simulink subsystem "algebraic_PIO_observer"  (R2024a)
settings: Solver=VariableStepAuto  StartTime=0.0  StopTime=10.0  RelTol=1e-3
undefined symbols (not defined in the file): Af, Cd, g, h, kf_A, kf_B, kf_C, kf_D, kf_L, l, lf, lr, M, re, rho_air
settings Model: Creator=Henrique Mesquita  LastModifiedBy=Henrique Mesquita
settings DebuggingCC: UnconnectedInputMsg=warning  UnconnectedOutputMsg=warning  UnconnectedLineMsg=warning
settings ModelReferenceCC: EnableRefExpFcnMdlSchedulingChecks=on
settings RTWCC: GPUComputeCapability=3.5  DLArmComputeVersion=19.05

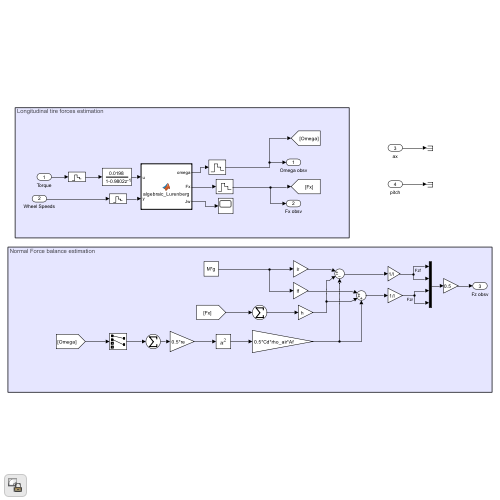
[thumbnail: Simulink's stored preview of the top-level diagram]
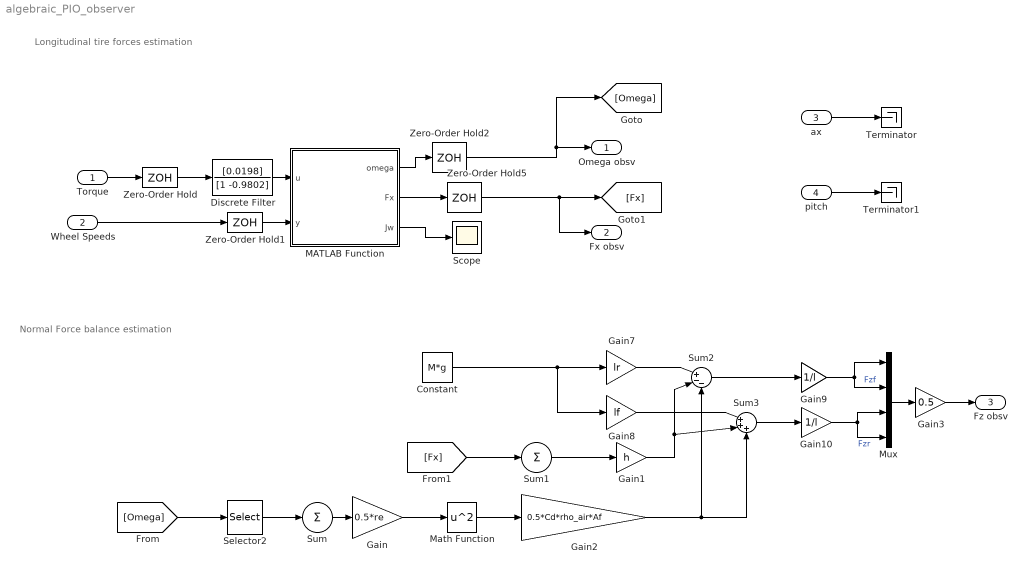
== system algebraic_PIO_observer ==
  note: Longitudinal tire forces estimation
  note: Normal Force balance estimation
  Torque : Inport  PortDimensions=4
  Wheel Speeds : Inport  Port=2  PortDimensions=4
  ax : Inport  Port=3  PortDimensions=1
  pitch : Inport  Port=4  PortDimensions=1
  Constant : Constant  Value=M*g
  Discrete Filter : DiscreteFilter  Numerator=[0.0198]  Denominator=[1 -0.9802]  SampleTime=0.001
  Gain : Gain  Gain=0.5*re
  Gain1 : Gain  Gain=h
  Gain10 : Gain  Gain=1/l
  Gain2 : Gain  Gain=0.5*Cd*rho_air*Af
  Gain3 : Gain  Gain=0.5
  Gain7 : Gain  Gain=lr
  Gain8 : Gain  Gain=lf
  Gain9 : Gain  Gain=1/l
  MATLAB Function : MATLAB Function  TreatAsAtomicUnit=on
  Math Function : Math  Operator=square
  Mux : Mux
  Scope : Scope
  Selector2 : Selector  InputPortWidth=4  IndexOptions=Index vector (dialog)  Indices=[1 2]  OutputSizes=1
  Sum : Sum  Inputs=+
  Sum1 : Sum  Inputs=+
  Sum2 : Sum  Inputs=|+--
  Sum3 : Sum  Inputs=|+++
  Terminator : Terminator
  Terminator1 : Terminator
  Zero-Order Hold{,1..2,5} (4 alike) : ZeroOrderHold  SampleTime=0.001
  Omega obsv : Outport
  Fx obsv : Outport  Port=2
  Fz obsv : Outport  Port=3
  wires:
  [Omega] -> Selector2/1
  Discrete Filter/1 -> MATLAB Function/1(u)
  Mux/1 -> Gain3/1
  Gain9/1 -> Mux/1, Mux/2  "Fzf"
  Gain2/1 -> Sum2/3, Sum3/3
  Gain1/1 -> Sum2/2, Sum3/2
  Gain3/1 -> Fz obsv/1
  Torque/1 -> Zero-Order Hold/1
  Constant/1 -> Gain7/1, Gain8/1
  Zero-Order Hold/1 -> Discrete Filter/1
  Gain/1 -> Math Function/1
  Math Function/1 -> Gain2/1
  Selector2/1 -> Sum/1
  [Fx] -> Sum1/1
  Gain7/1 -> Sum2/1
  Sum3/1 -> Gain10/1
  Gain10/1 -> Mux/3, Mux/4  "Fzr"
  MATLAB Function/1(omega) -> Zero-Order Hold2/1
  Zero-Order Hold2/1 -> Omega obsv/1, [Omega]
  Zero-Order Hold1/1 -> MATLAB Function/2(y)
  pitch/1 -> Terminator1/1
  Zero-Order Hold5/1 -> [Fx], Fx obsv/1
  Wheel Speeds/1 -> Zero-Order Hold1/1
  Gain8/1 -> Sum3/1
  ax/1 -> Terminator/1
  Sum2/1 -> Gain9/1
  Sum1/1 -> Gain1/1
  Sum/1 -> Gain/1
  MATLAB Function/2(Fx) -> Zero-Order Hold5/1
  MATLAB Function/3(Jw) -> Scope/1

== matlab function algebraic_PIO_observer/MATLAB Function ==
  data: u input size=4; y input size=4; omega output size=4; kf_L parameter; kf_A parameter; kf_B parameter; kf_C parameter; kf_D parameter; Fx output size=4; Jw output
function [omega, Fx, Jw] = algebraic_Lurenberg(u, y, kf_L, kf_A, kf_B, kf_C, kf_D)

N = 21;
Ts = 0.001;
Iw = 0.8;
alpha = 1/Iw;
re = 0.284;
% L = 1.25;

persistent xhat_ant;    % last state
persistent y_mem;       % last output
persistent u_mem;       % last input
persistent b0_ant;
persistent phi_ant;
persistent Fx_alg_ant;
persistent Fx_sso_ant;
persistent s_y;
persistent s_u;
persistent s_ay;
persistent s_au;

if(isempty(xhat_ant)||isempty(y_mem)||isempty(u_mem)||isempty(b0_ant)||isempty(phi_ant)||isempty(s_y)||isempty(s_u)||isempty(s_ay)||isempty(s_au))
    y_mem = zeros(4,N+1);
    u_mem = zeros(4,N+1);
    b0_ant = ones(1,1)/Iw;
    phi_ant = zeros(4,1);
    xhat_ant = zeros(8,1);
    Fx_alg_ant = zeros(4,1);
    Fx_sso_ant = zeros(4,1);
    
    %%% Early calculation and saving of the algebraic estimator coefficients
    T = N*Ts;
    i = N-1:-1:1;
    s_y = -6/T^3*[Ts/2*(T-2*N*Ts), Ts*(T-2*i*Ts), Ts/2*(T-2*0*Ts)];
    s_u = -6/T^3*[Ts/2*(T-N*Ts)*(N*Ts), Ts*(T-i*Ts).*(i*Ts), Ts/2*(T-0*Ts)*(0*Ts)];
    
    s_ay = [Ts/2*(T^2-6*T*N*Ts+6*(N*Ts)^2), Ts*(T^2-6*T*i*Ts+6*(i*Ts).^2), Ts/2*(T^2-6*T*0*Ts+6*(0*Ts)^2)];
    s_au = [Ts/2*(-T^2*N*Ts+3*T*(N*Ts)^2-2*(N*Ts)^3), Ts*(-T^2*i*Ts+3*T*(i*Ts).^2-2*(i*Ts).^3), Ts/2*0];

end

%%% Memory actualization
for i = 0:N-1
    u_mem(:,N+1-i) = u_mem(:,N-i);
    y_mem(:,N+1-i) = y_mem(:,N-i);
end
u_mem(:,1) = u;
y_mem(:,1) = y;

%%% Moment of Inertia Algebraic Estimation
b0_auxy=zeros(1,1);
b0_auxu=zeros(1,1);
for i=1:N+1
    b0_auxy = b0_auxy + s_ay(i)*y_mem(3,i);
    b0_auxu = b0_auxu + s_au(i)*u_mem(3,i);
end

if(abs(b0_auxu)<=1e-4)
    b0=b0_ant;
else
    b0=b0_auxy./b0_auxu;
end
Jw = 1./b0;

%%% Force Algebraic Estimation
phi=zeros(4,1);
for i=1:N+1
    phi = phi + s_y(i)*y_mem(:,i) + alpha*s_u(i)*u_mem(:,i);
end

% Fx = -Iw/re*phi;

% Prediction
xbar = kf_A*xhat_ant + kf_B*u;
% Correction
xhat = xbar + kf_L*(y-kf_C*xbar-kf_D*u);

omega = xhat(1:4);


% Fx_alg = 0.9512*Fx_alg_ant + 0.04877*(-Iw/re*phi_ant);          %Passa baixa
% Fx_sso = 0.9512*Fx_sso_ant + 0.9754*(xhat(5:8)-xhat_ant(5:8));  %Passa alta
% Fx = Fx_alg + Fx_sso;
Fx = (-Iw/re*phi + xhat(5:8))/2;

% Fx_alg_ant = Fx_alg;
% Fx_sso_ant = Fx_sso;
phi_ant=phi;
xhat_ant = xhat;
b0_ant = b0;
